simulink model "FSFB"  (R2022a)
settings: Solver=ode45  StartTime=0.0  StopTime=100  RelTol=1e-8  AbsTol=1e-8
values from neighbouring files (symbols this model uses):
  epsc = -epsc    [FEEDBACK_ODE.m]    (also in HW5.m = epsc2)
  etac = etac2    [HW5.m]
  I = diag([1200 2000 2800])    [HW5.m]
  kd = -kd    [HW5.m]
  kp = -kp    [HW5.m]
  X0 = [eps0;w0]    [HW5.m]
settings Model: Creator=Josh2  LastModifiedBy=Josh2

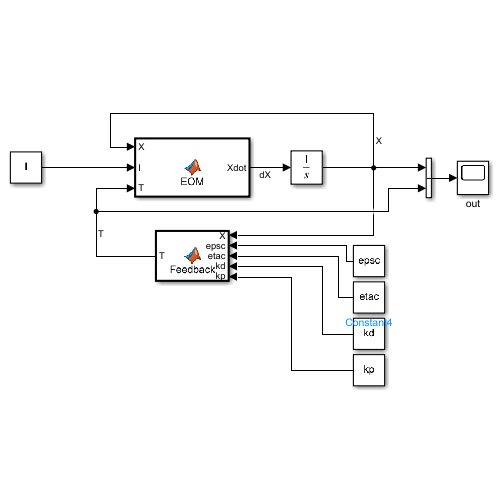
[thumbnail: Simulink's stored preview of the top-level diagram]
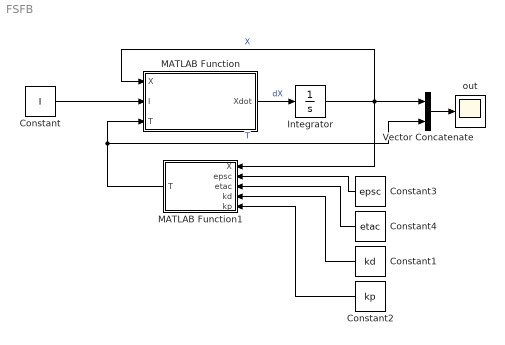
== system FSFB ==
  Constant : Constant  Value=I
  Constant1 : Constant  Value=kd
  Constant2 : Constant  Value=kp
  Constant3 : Constant  Value=epsc
  Constant4 : Constant  Value=etac
  Integrator : Integrator  InitialCondition=X0
  MATLAB Function : MATLAB Function  TreatAsAtomicUnit=on
  MATLAB Function1 : MATLAB Function  TreatAsAtomicUnit=on
  Vector Concatenate : Concatenate
  out : Scope
  wires:
  MATLAB Function/1(Xdot) -> Integrator/1  "dX"
  Integrator/1 -> MATLAB Function1/1(X), MATLAB Function/1(X), Vector Concatenate/1  "X"
  Constant/1 -> MATLAB Function/2(I)
  MATLAB Function1/1(T) -> MATLAB Function/3(T), Vector Concatenate/2  "T"
  Vector Concatenate/1 -> out/1
  Constant2/1 -> MATLAB Function1/5(kp)
  Constant1/1 -> MATLAB Function1/4(kd)
  Constant4/1 -> MATLAB Function1/3(etac)
  Constant3/1 -> MATLAB Function1/2(epsc)

== matlab function FSFB/MATLAB Function1 ==
  data: X input; T output; epsc input; etac input; kd input; kp input
function T = Feedback(X,epsc,etac,kd,kp)

% pass through for feedback function

T = zeros(3,1);
T = FEEDBACK_ODE(X,epsc,etac,kd,kp);
end

== matlab function FSFB/MATLAB Function ==
  data: Xdot output; X input; I input; T input
function Xdot = EOM(X,I,T)
% pass through function calls shared ODE (because this is the world we live in)
Xdot = zeros(10,1);
Xdot = EOM_ODE(0,X,I,T);
end
